simulink model "IfElse"  (R2020a)
settings: Solver=VariableStepAuto  StartTime=0.0  StopTime=10.0  RelTol=1e-3
settings Model: Creator=ashok  LastModifiedBy=ashok

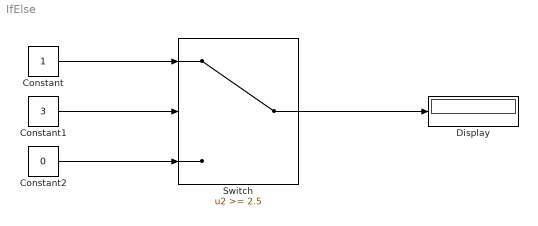
== system IfElse ==
  Constant : Constant
  Constant1 : Constant  Value=3
  Constant2 : Constant  Value=0
  Display : Display
  Switch : Switch  Threshold=2.5
  wires:
  Switch/1 -> Display/1
  Constant/1 -> Switch/1
  Constant1/1 -> Switch/2
  Constant2/1 -> Switch/3
